simulink model "AC_6DOF"  (R2021a)
settings: Solver=VariableStepAuto  StartTime=0.0  StopTime=25  RelTol=1e-3
model workspace (MAT data in the model file):
  J = [1  0.5  0.4; 0.5  1  0.6; 0.4  0.6  1]
  mass = 1
libraries: vrlib x3, aerolibutil x1, sharedutil x1
settings Model: OrderedModelArguments=off  Creator=davis  LastModifiedBy=dbradstr

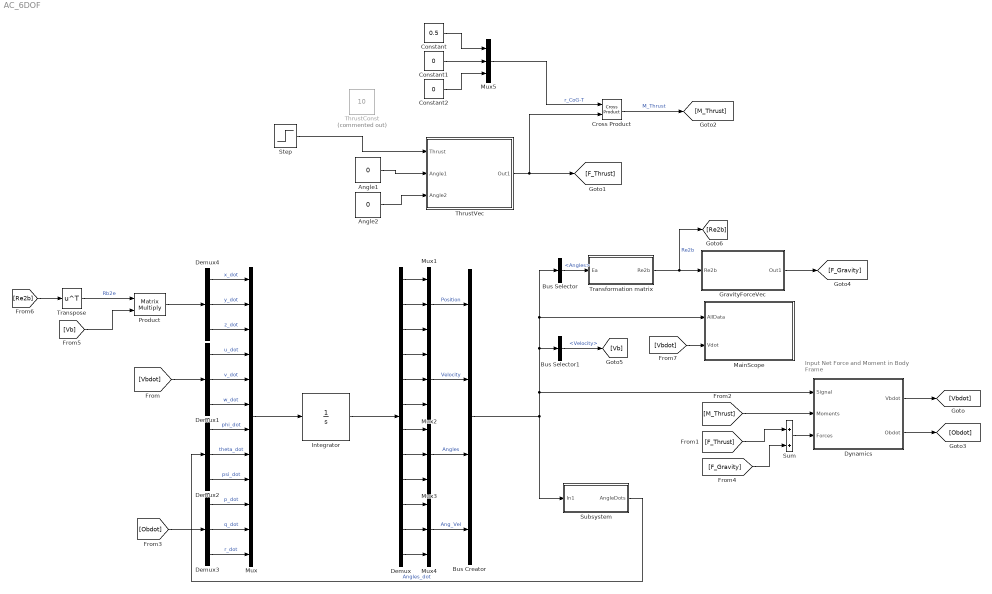
== system AC_6DOF ==
  note: Input Net Force and Moment in Body Frame
  Angle1 : Constant  Value=0
  Angle2 : Constant  Value=0
  Bus Creator : BusCreator  Inputs=4
  Bus Selector : BusSelector  OutputSignals=Angles
  Bus Selector1 : BusSelector  OutputSignals=Velocity
  Constant : Constant  Value=0.5
  Constant1 : Constant  Value=0
  Constant2 : Constant  Value=0
  Cross Product : vrlib/Utilities/Cross Product
  Demux : Demux  Outputs=12
  Demux{1..4} (4 alike) : Demux  Outputs=3
  Dynamics : Subsystem
  GravityForceVec : Subsystem
  Integrator : Integrator
  MainScope : Subsystem
  Mux : Mux  Inputs=12
  Mux{1..5} (5 alike) : Mux  Inputs=3
  Product : Product  Multiplication=Matrix(*)
  Step : Step  Time=3  Before=30  After=0  SampleTime=0
  Subsystem : Subsystem
  Sum : Sum  Inputs=|++
  ThrustConst : Constant  Commented=on  Value=10
  ThrustVec : Subsystem
  Transformation matrix : Subsystem
  Transpose : Math  Operator=transpose  SaturateOnIntegerOverflow=on
  wires:
  Mux/1 -> Integrator/1
  Integrator/1 -> Demux/1
  Demux/3 -> Mux1/3
  Demux/2 -> Mux1/2
  Demux/1 -> Mux1/1
  Mux1/1 -> Bus Creator/1  "Position"
  Mux2/1 -> Bus Creator/2  "Velocity"
  Demux/4 -> Mux2/1
  Demux/5 -> Mux2/2
  Demux/6 -> Mux2/3
  Mux3/1 -> Bus Creator/3  "Angles"
  Demux/7 -> Mux3/1
  Demux/8 -> Mux3/2
  Demux/9 -> Mux3/3
  Mux4/1 -> Bus Creator/4  "Ang_Vel"
  Demux/10 -> Mux4/1
  Demux/11 -> Mux4/2
  Demux/12 -> Mux4/3
  Bus Creator/1 -> Subsystem/1(In1), Dynamics/1(Signal), Bus Selector1/1, Bus Selector/1, MainScope/1(AllData)
  Bus Selector/1 -> Transformation matrix/1(Ea)  "<Angles>"
  Demux1/1 -> Mux/4  "u_dot"
  Demux1/2 -> Mux/5  "v_dot"
  Demux1/3 -> Mux/6  "w_dot"
  Dynamics/1(Vbdot) -> [Vbdot]
  [Vbdot] -> Demux1/1
  Constant2/1 -> Mux5/3
  Constant1/1 -> Mux5/2
  Constant/1 -> Mux5/1
  Mux5/1 -> Cross Product/1  "r_CoG-T"
  Angle1/1 -> ThrustVec/2(Angle1)
  Angle2/1 -> ThrustVec/3(Angle2)
  ThrustVec/1(Out1) -> [F_Thrust], Cross Product/2
  Cross Product/1 -> [M_Thrust]  "M_Thrust"
  Subsystem/1(AngleDots) -> Demux2/1  "Angles_dot"
  Demux2/3 -> Mux/9  "psi_dot"
  Demux2/2 -> Mux/8  "theta_dot"
  Demux2/1 -> Mux/7  "phi_dot"
  [M_Thrust] -> Dynamics/2(Moments)
  Dynamics/2(Obdot) -> [Obdot]
  Demux3/1 -> Mux/10  "p_dot"
  Demux3/2 -> Mux/11  "q_dot"
  Demux3/3 -> Mux/12  "r_dot"
  [Obdot] -> Demux3/1
  Sum/1 -> Dynamics/3(Forces)
  [F_Thrust] -> Sum/1
  [F_Gravity] -> Sum/2
  Transformation matrix/1(Re2b) -> [Re2b], GravityForceVec/1(Re2b)  "Re2b"
  GravityForceVec/1(Out1) -> [F_Gravity]
  Bus Selector1/1 -> [Vb]  "<Velocity>"
  [Re2b] -> Transpose/1
  Transpose/1 -> Product/1  "Rb2e"
  [Vb] -> Product/2
  Demux4/1 -> Mux/1  "x_dot"
  Demux4/2 -> Mux/2  "y_dot"
  Demux4/3 -> Mux/3  "z_dot"
  Product/1 -> Demux4/1
  Step/1 -> ThrustVec/1(Thrust)
  [Vbdot] -> MainScope/2(Vdot)

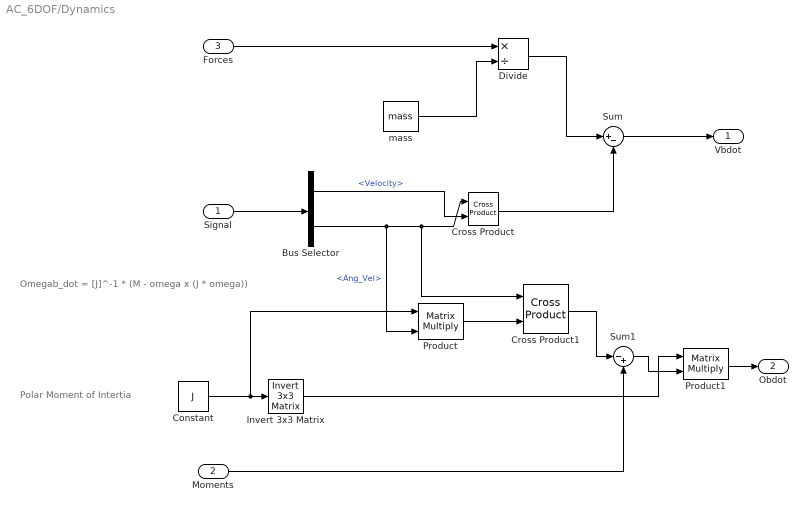
== system AC_6DOF/Dynamics ==
  note: Omegab_dot = [J]^-1 * (M - omega x (J * omega))
  note: Polar Moment of Intertia
  Signal : Inport
  Moments : Inport  Port=2
  Forces : Inport  Port=3
  Bus Selector : BusSelector  OutputSignals=Velocity,Ang_Vel
  Constant : Constant  Value=J
  Cross Product : vrlib/Utilities/Cross Product
  Cross Product1 : vrlib/Utilities/Cross Product
  Divide : Product  Inputs=*/
  Invert 3x3 Matrix : aerolibutil/Invert  3x3 Matrix
  Product : Product  Multiplication=Matrix(*)
  Product1 : Product  Multiplication=Matrix(*)
  Sum : Sum  Inputs=|+-
  Sum1 : Sum  Inputs=|-+
  mass : Constant  Value=mass
  Vbdot : Outport
  Obdot : Outport  Port=2
  wires:
  mass/1 -> Divide/2
  Signal/1 -> Bus Selector/1
  Forces/1 -> Divide/1
  Bus Selector/1 -> Cross Product/2  "<Velocity>"
  Bus Selector/2 -> Product/2, Cross Product1/1, Cross Product/1  "<Ang_Vel>"
  Divide/1 -> Sum/1
  Cross Product/1 -> Sum/2
  Sum/1 -> Vbdot/1
  Constant/1 -> Product/1, Invert 3x3 Matrix/1
  Invert 3x3 Matrix/1 -> Product1/1
  Product/1 -> Cross Product1/2
  Moments/1 -> Sum1/2
  Cross Product1/1 -> Sum1/1
  Sum1/1 -> Product1/2
  Product1/1 -> Obdot/1

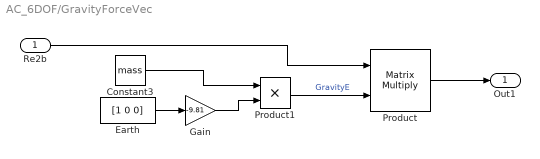
== system AC_6DOF/GravityForceVec ==
  Re2b : Inport
  Constant3 : Constant  Value=mass
  Earth : Constant  Value=[1 0 0]
  Gain : Gain  Gain=-9.81
  Product : Product  Multiplication=Matrix(*)
  Product1 : Product
  Out1 : Outport
  wires:
  Product/1 -> Out1/1
  Re2b/1 -> Product/1
  Earth/1 -> Gain/1
  Gain/1 -> Product1/2
  Product1/1 -> Product/2  "GravityE"
  Constant3/1 -> Product1/1

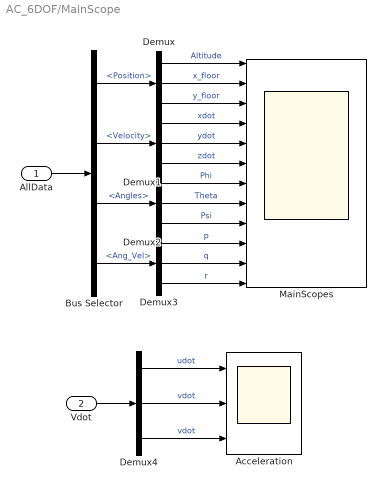
== system AC_6DOF/MainScope ==
  AllData : Inport
  Vdot : Inport  Port=2
  Acceleration : Scope  NumInputPorts=3
  Bus Selector : BusSelector  OutputSignals=Position,Velocity,Angles,Ang_Vel
  Demux{,1..4} (5 alike) : Demux  Outputs=3
  MainScopes : Scope  NumInputPorts=12
  wires:
  Bus Selector/1 -> Demux/1  "<Position>"
  Demux/1 -> MainScopes/1  "Altitude"
  Demux/2 -> MainScopes/2  "x_floor"
  Demux/3 -> MainScopes/3  "y_floor"
  Demux1/3 -> MainScopes/6  "zdot"
  Demux1/1 -> MainScopes/4  "xdot"
  Demux1/2 -> MainScopes/5  "ydot"
  Bus Selector/2 -> Demux1/1  "<Velocity>"
  Demux2/3 -> MainScopes/9  "Psi"
  Demux2/1 -> MainScopes/7  "Phi"
  Demux3/2 -> MainScopes/11  "q"
  Demux2/2 -> MainScopes/8  "Theta"
  Bus Selector/3 -> Demux2/1  "<Angles>"
  Demux3/3 -> MainScopes/12  "r"
  Bus Selector/4 -> Demux3/1  "<Ang_Vel>"
  Demux3/1 -> MainScopes/10  "p"
  AllData/1 -> Bus Selector/1
  Demux4/2 -> Acceleration/2  "vdot"
  Demux4/1 -> Acceleration/1  "udot"
  Demux4/3 -> Acceleration/3  "vdot"
  Vdot/1 -> Demux4/1

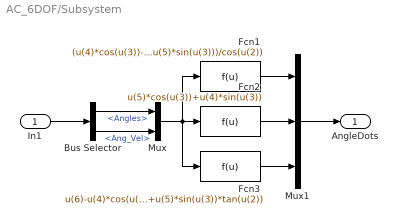
== system AC_6DOF/Subsystem ==
  In1 : Inport
  Bus Selector : BusSelector  OutputSignals=Angles,Ang_Vel
  Fcn1 : Fcn  Expr=(u(4)*cos(u(3))-u(5)*sin(u(3)))/cos(u(2))
  Fcn2 : Fcn  Expr=u(5)*cos(u(3))+u(4)*sin(u(3))
  Fcn3 : Fcn  Expr=u(6)-u(4)*cos(u(3))*tan(u(2))+u(5)*sin(u(3))*tan(u(2))
  Mux : Mux  Inputs=2
  Mux1 : Mux  Inputs=3
  AngleDots : Outport
  wires:
  In1/1 -> Bus Selector/1
  Bus Selector/1 -> Mux/1  "<Angles>"
  Bus Selector/2 -> Mux/2  "<Ang_Vel>"
  Mux/1 -> Fcn2/1, Fcn3/1, Fcn1/1
  Fcn2/1 -> Mux1/2
  Fcn1/1 -> Mux1/1
  Fcn3/1 -> Mux1/3
  Mux1/1 -> AngleDots/1

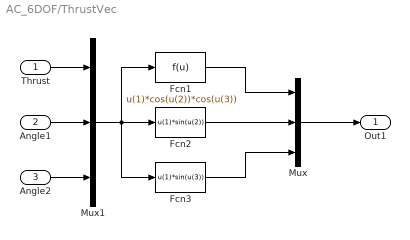
== system AC_6DOF/ThrustVec ==
  Thrust : Inport
  Angle1 : Inport  Port=2
  Angle2 : Inport  Port=3
  Fcn1 : Fcn  Expr=u(1)*cos(u(2))*cos(u(3))
  Fcn2 : Fcn  Expr=u(1)*sin(u(2))
  Fcn3 : Fcn  Expr=u(1)*sin(u(3))
  Mux : Mux  Inputs=3
  Mux1 : Mux  Inputs=3
  Out1 : Outport
  wires:
  Mux/1 -> Out1/1
  Angle2/1 -> Mux1/3
  Angle1/1 -> Mux1/2
  Thrust/1 -> Mux1/1
  Mux1/1 -> Fcn1/1, Fcn2/1, Fcn3/1
  Fcn2/1 -> Mux/2
  Fcn1/1 -> Mux/1
  Fcn3/1 -> Mux/3

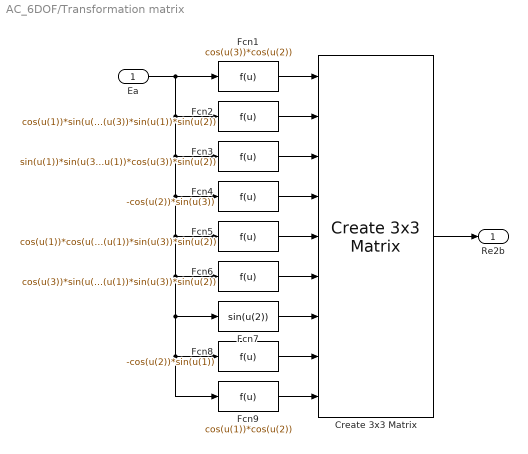
== system AC_6DOF/Transformation matrix ==
  Ea : Inport
  Create 3x3 Matrix : sharedutil/Create 3x3 Matrix  aMode=aMode
      settings: SourceProductBaseCode=AE,PW,MT,UV,VE,VP
  Fcn1 : Fcn  Expr=cos(u(3))*cos(u(2))
  Fcn2 : Fcn  Expr=cos(u(1))*sin(u(3)) + cos(u(3))*sin(u(1))*sin(u(2))
  Fcn3 : Fcn  Expr=sin(u(1))*sin(u(3)) - cos(u(1))*cos(u(3))*sin(u(2))
  Fcn4 : Fcn  Expr=-cos(u(2))*sin(u(3))
  Fcn5 : Fcn  Expr=cos(u(1))*cos(u(3)) - sin(u(1))*sin(u(3))*sin(u(2))
  Fcn6 : Fcn  Expr=cos(u(3))*sin(u(1)) + cos(u(1))*sin(u(3))*sin(u(2))
  Fcn7 : Fcn  Expr=sin(u(2))
  Fcn8 : Fcn  Expr=-cos(u(2))*sin(u(1))
  Fcn9 : Fcn  Expr=cos(u(1))*cos(u(2))
  Re2b : Outport  VectorParamsAs1DForOutWhenUnconnected=off
  wires:
  Ea/1 -> Fcn9/1, Fcn8/1, Fcn7/1, Fcn6/1, Fcn5/1, Fcn4/1, Fcn3/1, Fcn2/1, Fcn1/1
  Fcn9/1 -> Create 3x3 Matrix/9
  Fcn8/1 -> Create 3x3 Matrix/8
  Fcn7/1 -> Create 3x3 Matrix/7
  Fcn6/1 -> Create 3x3 Matrix/6
  Fcn5/1 -> Create 3x3 Matrix/5
  Fcn4/1 -> Create 3x3 Matrix/4
  Fcn3/1 -> Create 3x3 Matrix/3
  Fcn2/1 -> Create 3x3 Matrix/2
  Fcn1/1 -> Create 3x3 Matrix/1
  Create 3x3 Matrix/1 -> Re2b/1
